simulink model "IRFsdof"  (R2015a)
settings: Solver=ode45  StartTime=0.0  StopTime=10.0  RelTol=1e-3
values from neighbouring files (symbols this model uses):
  k = 1000/3    (= 333.333333333)    [can2v.m]
undefined symbols (not defined in the file or in its folder): c, m
settings Model: Creator=USER  LastModifiedBy=USER

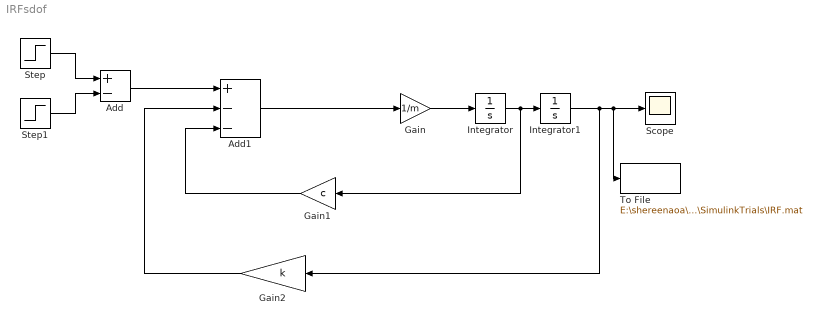
== system IRFsdof ==
  Add : Sum  Inputs=+-
  Add1 : Sum  Inputs=+--
  Gain : Gain  Gain=1/m
  Gain1 : Gain  Gain=c
  Gain2 : Gain  Gain=k
  Integrator : Integrator
  Integrator1 : Integrator
  Scope : Scope
  Step : Step  Time=0  After=0.2  SampleTime=0.2
  Step1 : Step  Time=5  After=0.2  SampleTime=0.2
  To File : ToFile  Filename=E:\shereenaoa\MyD\MATLABCodz\Mycodz\SimulinkTrials\IRF.mat  MatrixName=irf
  wires:
  Step/1 -> Add/1
  Step1/1 -> Add/2
  Add/1 -> Add1/1
  Gain2/1 -> Add1/2
  Gain1/1 -> Add1/3
  Add1/1 -> Gain/1
  Gain/1 -> Integrator/1
  Integrator/1 -> Gain1/1, Integrator1/1
  Integrator1/1 -> Gain2/1, To File/1, Scope/1
